simulink model "PPS_COM"  (R2022b)
settings: configuration reference "PPS_AutosarConfig" (kept outside this file)
model workspace (MATLAB code in the model file):
  | cmdLim = Simulink.Parameter;
  | cmdLim.Value = 15;
  | cmdLim.Description = 'Limit for controlling the maximum surface command angle.';
  | cmdLim.Min = 0;
  | cmdLim.Max = 90;
  | cmdLim.DocUnits = 'deg';
  | 
  | dispGain = Simulink.Parameter;
  | dispGain.Value = 0.75;
  | dispGain.Description = 'Gain applied to the displacement error.';
  | dispGain.Min = 0;
  | dispGain.Max = [];
  | dispGain.DocUnits = 'deg/sec/deg';
  | 
  | dispLim = Simulink.Parameter;
  | dispLim.Value = 30;
  | dispLim.Description = 'Limit for controlling the maximum commanded angle.';
  | dispLim.Min = 0;
  | dispLim.Max = 180;
  | dispLim.DocUnits = 'deg';
  | 
  | intGain = Simulink.Parameter;
  | intGain.Value = 0.5;
  | intGain.Description = 'Gain applied to the integral error.';
  | intGain.Min = 0;
  | intGain.Max = [];
  | intGain.DocUnits = 'deg/sec/deg/sec';
  | 
  | intLim = Simulink.Parameter;
  | intLim.Value = 5;
  | intLim.Description = 'Limit for controlling the maximum commanded angle.';
  | intLim.Min = 0;
  | intLim.Max = 90;
  | intLim.DocUnits = 'deg';
  | 
  | rateGain = Simulink.Parameter;
  | rateGain.Value = 2;
  | rateGain.Description = 'Gain applied to the rate error.';
  | rateGain.Min = 0;
  | rateGain.Max = [];
  | rateGain.DocUnits = 'deg/deg/sec';
  | 
  | rateLim = Simulink.Parameter;
  | rateLim.Value = 6;
  | rateLim.Description = 'Limit for controlling the maximum commanded angle.';
  | rateLim.Min = 0;
  | rateLim.Max = 180;
  | rateLim.DocUnits = 'deg/sec';
  | 
  | hdgGain = Simulink.Parameter;
  | hdgGain.Value = 0.015;
values from neighbouring files (symbols this model uses):
  PPS_SampleTime = 0.01    [PPS_DD.sldd]
settings Model: RequirementInfo={} %GIDa_fe9045fd_0412_4b6e_8206_617cc20e6fde  DataDictionary=PPS_DD.sldd  FPTRunName=Active  Creator=MAAM  LastModifiedBy=MAAM
settings ConfigSetRef: SourceName=PPS_AutosarConfig

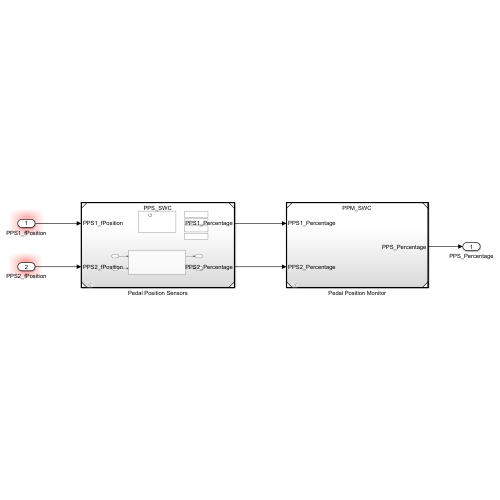
[thumbnail: Simulink's stored preview of the top-level diagram]
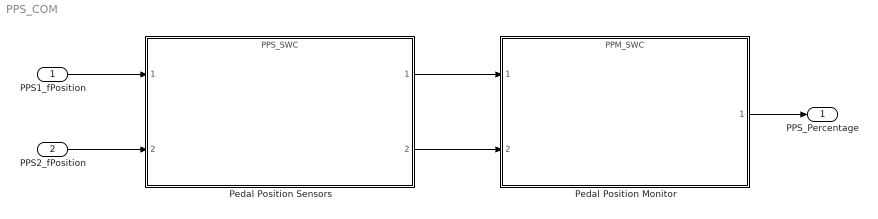
== system PPS_COM ==
  PPS1_fPosition : Inport  OutDataTypeStr=uint16  SampleTime=PPS_SampleTime
  PPS2_fPosition : Inport  Port=2  OutDataTypeStr=uint16  SampleTime=PPS_SampleTime
  Pedal Position Monitor : ModelReference  ModelNameDialog=PPM_SWC  SimulationMode=Normal  ModelReferenceVersion=1.2
  Pedal Position Sensors : ModelReference  ModelNameDialog=PPS_SWC  SimulationMode=Normal  ModelReferenceVersion=1.6
  PPS_Percentage : Outport
  wires:
  Pedal Position Sensors/1 -> Pedal Position Monitor/1
  Pedal Position Sensors/2 -> Pedal Position Monitor/2
  PPS1_fPosition/1 -> Pedal Position Sensors/1
  PPS2_fPosition/1 -> Pedal Position Sensors/2
  Pedal Position Monitor/1 -> PPS_Percentage/1
